simulink model "example_rotor_MRAC"  (R2016a)
settings: Solver=VariableStepAuto  StartTime=0.0  StopTime=30  RelTol=1e-3
values from neighbouring files (symbols this model uses):
  load_amp = 1    [configuration.mat]
  load_finish = 22    [configuration.mat]
  load_start = 10    [configuration.mat]
  measurement_variance = 15    [configuration.mat]
  MRACparam =     [configuration.mat]
  pulse_period = 8    [configuration.mat]
  ref_amp = 200    [configuration.mat]
  ref_mean = 2000    [configuration.mat]
  rotor_h = 0.002    [configuration.mat]
  sinusoid_frequency = 1    [configuration.mat]
settings Model: Creator=mgreiff  LastModifiedBy=mgreiff

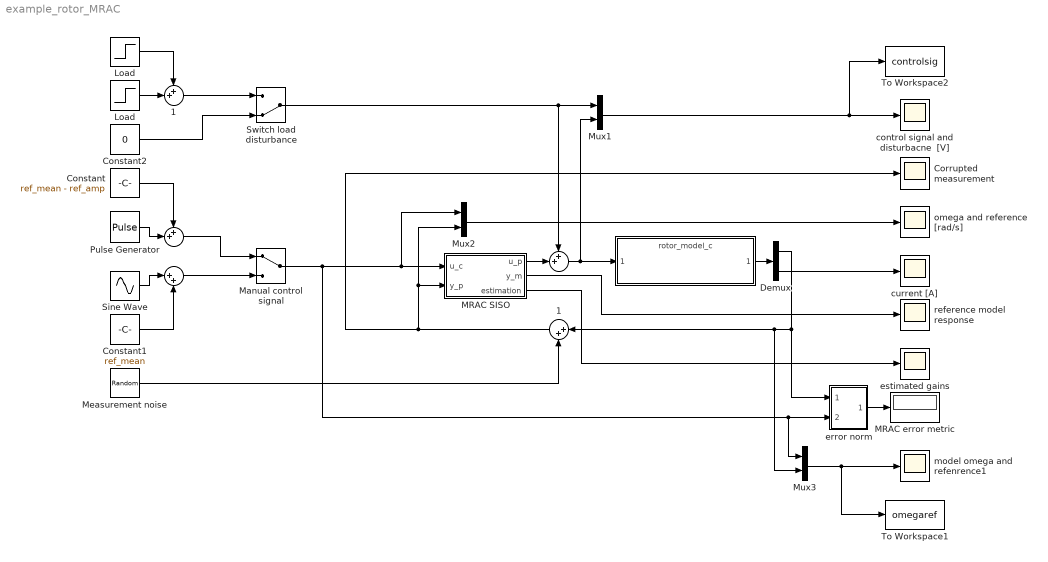
== system example_rotor_MRAC ==
  " " : Sum  Inputs=++|
  "   " : ModelReference  ModelNameDialog=rotor_model_c.slx  SimulationMode=Normal  ModelReferenceVersion=1.30
  "      " : Sum  Inputs=++|
  "       " : Sum  Inputs=|++
  "       1" : Sum  Inputs=|++
  "      1" : Sum  Inputs=++|
  " omega and reference [rad/s]" : Scope
  Constant : Constant  Value=ref_mean - ref_amp
  Constant1 : Constant  Value=ref_mean
  Constant2 : Constant  Value=0
  Corrupted measurement : Scope
  Demux : Demux  Outputs=2
  Load : Step  Time=load_finish  After=-load_amp  SampleTime=0
  "Load " : Step  Time=load_start  After=load_amp  SampleTime=0
  MRAC SISO : Subsystem
  MRAC error metric : Display
  Manual control signal : ManualSwitch
  Measurement noise : RandomNumber  Variance=measurement_variance  SampleTime=rotor_h
  Mux1 : Mux  Inputs=2
  Mux2 : Mux  Inputs=2
  Mux3 : Mux  Inputs=2
  Pulse Generator : DiscretePulseGenerator  PulseType=Time based  Amplitude=ref_amp*2  Period=pulse_period  PulseWidth=50
  Sine Wave : Sin  Amplitude=200  Frequency=sinusoid_frequency  SampleTime=0
  Switch load disturbance : ManualSwitch  CurrentSetting=0
  To Workspace1 : ToWorkspace  VariableName=omegaref  SaveFormat=Timeseries  SampleTime=-1
  To Workspace2 : ToWorkspace  VariableName=controlsig  SaveFormat=Timeseries  SampleTime=-1
  control signal and disturbacne  [V] : Scope
  "current [A]   " : Scope
  error norm : Subsystem
  estimated gains : Scope
  model omega and refenrence1 : Scope
  reference model response : Scope
  wires:
  "   "/1 -> Demux/1
  Constant/1 -> "      "/1
  Demux/2 -> "current [A]   "/1
  "      "/1 -> Manual control signal/1
  Pulse Generator/1 -> "      "/2
  Sine Wave/1 -> "       "/1
  "       "/1 -> Manual control signal/2
  Constant1/1 -> "       "/2
  " "/1 -> Mux1/2, "   "/1
  Manual control signal/1 -> error norm/2(In2), Mux3/1, MRAC SISO/1(u_c), Mux2/1
  Switch load disturbance/1 -> " "/1, Mux1/1
  Mux1/1 -> To Workspace2/1, control signal and disturbacne  [V]/1
  Mux3/1 -> To Workspace1/1, model omega and refenrence1/1
  "Load "/1 -> "      1"/1
  Load/1 -> "      1"/2
  error norm/1(Out1) -> MRAC error metric/1
  "      1"/1 -> Switch load disturbance/1
  Constant2/1 -> Switch load disturbance/2
  Demux/1 -> "       1"/1, Mux3/2, error norm/1(In1)
  "       1"/1 -> MRAC SISO/2(y_p), Mux2/2, Corrupted measurement/1
  Measurement noise/1 -> "       1"/2
  MRAC SISO/1(u_p) -> " "/2
  MRAC SISO/3(estimation) -> estimated gains/1
  MRAC SISO/2(y_m) -> reference model response/1
  Mux2/1 -> " omega and reference [rad/s]"/1

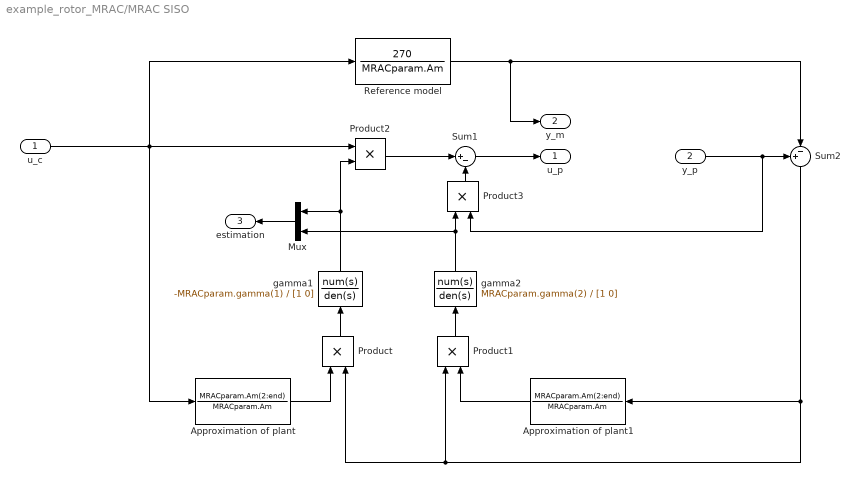
== system example_rotor_MRAC/MRAC SISO ==
  u_c : Inport
  y_p : Inport  Port=2
  " gamma2" : TransferFcn  Numerator=MRACparam.gamma(2)  Denominator=[1 0]
  Approximation of plant : TransferFcn  Numerator=MRACparam.Am(2:end)  Denominator=MRACparam.Am
  Approximation of plant1 : TransferFcn  Numerator=MRACparam.Am(2:end)  Denominator=MRACparam.Am
  Mux : Mux  Inputs=2
  Product{,1..3} (4 alike) : Product
  Reference model : TransferFcn  Numerator=270  Denominator=MRACparam.Am
  Sum1 : Sum  Inputs=|+-
  Sum2 : Sum  Inputs=+-|
  gamma1 : TransferFcn  Numerator=-MRACparam.gamma(1)  Denominator=[1 0]
  u_p : Outport
  y_m : Outport  Port=2
  estimation : Outport  Port=3
  wires:
  Sum1/1 -> u_p/1
  gamma1/1 -> Product2/2, Mux/1
  " gamma2"/1 -> Mux/2, Product3/1
  y_p/1 -> Sum2/1, Product3/2
  Approximation of plant/1 -> Product/1
  Product1/1 -> " gamma2"/1
  Sum2/1 -> Approximation of plant1/1, Product1/1, Product/2
  Product2/1 -> Sum1/1
  Approximation of plant1/1 -> Product1/2
  u_c/1 -> Approximation of plant/1, Product2/1, Reference model/1
  Product3/1 -> Sum1/2
  Product/1 -> gamma1/1
  Reference model/1 -> y_m/1, Sum2/2
  Mux/1 -> estimation/1

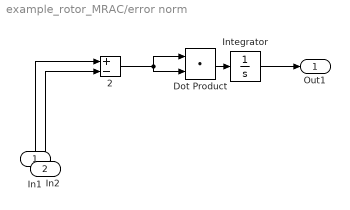
== system example_rotor_MRAC/error norm ==
  In1 : Inport
  In2 : Inport  Port=2
  "      2" : Sum  Inputs=+-
  Dot Product : DotProduct  InputSameDT=on  OutDataTypeStr=Inherit: Inherit via internal rule
  Integrator : Integrator
  Out1 : Outport
  wires:
  "      2"/1 -> Dot Product/1, Dot Product/2
  Dot Product/1 -> Integrator/1
  In1/1 -> "      2"/1
  In2/1 -> "      2"/2
  Integrator/1 -> Out1/1
